simulink model "Adaptive_flux_observer_with_rotor_resistance_estimator"  (R2021a)
settings: Solver=FixedStepDiscrete  StartTime=0.0  StopTime=10.0  FixedStep=1e-5  RelTol=1e-3
undefined symbols (not defined in the file): DiscIntNeverNeededParam
settings Model: Creator=Mehra  LastModifiedBy=Mehra
settings SolverCC: ZeroCrossControl=DisableAll
settings DataIOCC: SaveOutput=off  SaveTime=off
settings GRTTargetCC: CombineOutputUpdateFcns=off  MatFileLogging=off

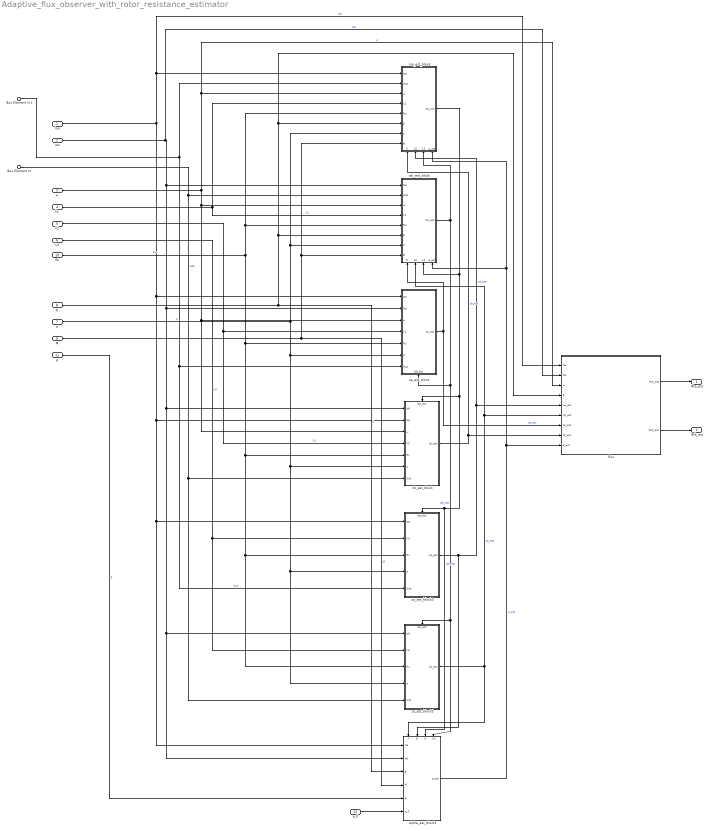
== system Adaptive_flux_observer_with_rotor_resistance_estimator ==
  Isa : Inport
  Isb : Inport  Port=2
  ω : Inport  Port=3
  k1 : Inport  Port=4
  k2 : Inport  Port=5
  k3 : Inport  Port=6
  σ : Inport  Port=7  OutDataTypeStr=double  PortDimensions=1
  β : Inport  Port=8  OutDataTypeStr=double  PortDimensions=1
  M : Inport  Port=9  OutDataTypeStr=double  PortDimensions=1
  Rs : Inport  Port=10
  g : Inport  Port=11
  α_0 : Inport  Port=12
  Bus Element In : Inport  Port=13  PortName=Uab  Element=Usb
  Bus Element In1 : Inport  Port=13  PortName=Uab  Element=Usa
  Isb_est_block : Subsystem
      settings: PortSchema="{\"entries\":[{\"content\":{\"sides\":[{\"content\":{\"connectorIds\":[\"In1\",\"In2\",\"In3\",\"In4\",\"In5\",\"In6\",\"In7\",\"In8\"]},\"type\":\"ConnectorPlacement.EquallySpacedRectSide\",\"uuid\":\"87550367-2c6c-480a-aae3-af00ec1c69b3\"},{\"content\":{\"connectorIds\":[\"Out1\"],\"side\":\"RIGHT\"},\"type\":\"ConnectorPlacement.EquallySpacedRectSide\",\"uuid\":\"4f526c6d-fa4b-4ae0-86ac-8e6f33c5fae1\"},{\"content\":{\"connectorIds\":[],\"side\":\"TOP\"},\"type\":\"ConnectorPlacement.EquallySpacedRectSide\",\"uuid\":\"2d7b9d3a-1034-4362-9035-011a628f41c9\"},{\"content\":{\"connectorIds\":[\"In9\",\"In10\",\"In11\",\"In12\"],\"side\":\"BOTTOM\"},\"type\":\"ConnectorPlacement.EquallySpacedRectSide\",\"uuid\":\"27bebb74-37d6-4f42-a6d1-29615f974c06\"}]},\"type\":\"ConnectorPlacement.EquallySpacedConnector\",\"uuid\":\"0c2c7644-fd75-4008-b344-0d549d52e423\"}],\"packageUris\":[\"http://schema.mathworks.com/mf0/Connector/R2020b\"],\"version\":\"1.0\"}"
  alpha_est_block1 : Subsystem
      settings: PortSchema="{\"entries\":[{\"content\":{\"sides\":[{\"content\":{\"connectorIds\":[\"In1\",\"In2\",\"In3\",\"In4\",\"In5\",\"In6\"]},\"type\":\"ConnectorPlacement.EquallySpacedRectSide\",\"uuid\":\"13ad627c-6f07-4cec-b595-5beaa6b2cc7c\"},{\"content\":{\"connectorIds\":[\"Out1\"],\"side\":\"RIGHT\"},\"type\":\"ConnectorPlacement.EquallySpacedRectSide\",\"uuid\":\"277076a7-856b-4e3b-b26b-d287057d48dc\"},{\"content\":{\"connectorIds\":[\"In7\",\"In8\",\"In9\",\"In10\"],\"side\":\"TOP\"},\"type\":\"ConnectorPlacement.EquallySpacedRectSide\",\"uuid\":\"ff90b138-b04e-44ba-87a2-7f09928b1812\"},{\"content\":{\"connectorIds\":[],\"side\":\"BOTTOM\"},\"type\":\"ConnectorPlacement.EquallySpacedRectSide\",\"uuid\":\"47c98a3f-b8ed-4eae-8b18-f11cd62e73ac\"}]},\"type\":\"ConnectorPlacement.EquallySpacedConnector\",\"uuid\":\"bcf44069-4ce9-4b3f-954c-53de8c0b8283\"}],\"packageUris\":[\"http://schema.mathworks.com/mf0/Connector/R2020b\"],\"version\":\"1.0\"}"
  flux : Subsystem
  isa_est_block : Subsystem
      settings: PortSchema="{\"entries\":[{\"content\":{\"sides\":[{\"content\":{\"connectorIds\":[\"In1\",\"In2\",\"In3\",\"In4\",\"In5\",\"In6\",\"In7\",\"In8\"]},\"type\":\"ConnectorPlacement.EquallySpacedRectSide\",\"uuid\":\"87550367-2c6c-480a-aae3-af00ec1c69b3\"},{\"content\":{\"connectorIds\":[\"Out1\"],\"side\":\"RIGHT\"},\"type\":\"ConnectorPlacement.EquallySpacedRectSide\",\"uuid\":\"4f526c6d-fa4b-4ae0-86ac-8e6f33c5fae1\"},{\"content\":{\"connectorIds\":[],\"side\":\"TOP\"},\"type\":\"ConnectorPlacement.EquallySpacedRectSide\",\"uuid\":\"2d7b9d3a-1034-4362-9035-011a628f41c9\"},{\"content\":{\"connectorIds\":[\"In9\",\"In10\",\"In11\",\"In12\"],\"side\":\"BOTTOM\"},\"type\":\"ConnectorPlacement.EquallySpacedRectSide\",\"uuid\":\"27bebb74-37d6-4f42-a6d1-29615f974c06\"}]},\"type\":\"ConnectorPlacement.EquallySpacedConnector\",\"uuid\":\"0c2c7644-fd75-4008-b344-0d549d52e423\"}],\"packageUris\":[\"http://schema.mathworks.com/mf0/Connector/R2020b\"],\"version\":\"1.0\"}"
  za_est_block : Subsystem
      settings: PortSchema="{\"entries\":[{\"content\":{\"sides\":[{\"content\":{\"connectorIds\":[\"In1\",\"In2\",\"In3\",\"In4\",\"In5\",\"In6\",\"In7\"]},\"type\":\"ConnectorPlacement.EquallySpacedRectSide\",\"uuid\":\"13ad627c-6f07-4cec-b595-5beaa6b2cc7c\"},{\"content\":{\"connectorIds\":[\"Out1\"],\"side\":\"RIGHT\"},\"type\":\"ConnectorPlacement.EquallySpacedRectSide\",\"uuid\":\"277076a7-856b-4e3b-b26b-d287057d48dc\"},{\"content\":{\"connectorIds\":[],\"side\":\"TOP\"},\"type\":\"ConnectorPlacement.EquallySpacedRectSide\",\"uuid\":\"ff90b138-b04e-44ba-87a2-7f09928b1812\"},{\"content\":{\"connectorIds\":[\"In8\"],\"side\":\"BOTTOM\"},\"type\":\"ConnectorPlacement.EquallySpacedRectSide\",\"uuid\":\"47c98a3f-b8ed-4eae-8b18-f11cd62e73ac\"}]},\"type\":\"ConnectorPlacement.EquallySpacedConnector\",\"uuid\":\"bcf44069-4ce9-4b3f-954c-53de8c0b8283\"}],\"packageUris\":[\"http://schema.mathworks.com/mf0/Connector/R2020b\"],\"version\":\"1.0\"}"
  za_est_block2 : Subsystem
      settings: PortSchema="{\"entries\":[{\"content\":{\"sides\":[{\"content\":{\"connectorIds\":[\"In1\",\"In2\",\"In3\",\"In4\",\"In5\"]},\"type\":\"ConnectorPlacement.EquallySpacedRectSide\",\"uuid\":\"13ad627c-6f07-4cec-b595-5beaa6b2cc7c\"},{\"content\":{\"connectorIds\":[\"Out1\"],\"side\":\"RIGHT\"},\"type\":\"ConnectorPlacement.EquallySpacedRectSide\",\"uuid\":\"277076a7-856b-4e3b-b26b-d287057d48dc\"},{\"content\":{\"connectorIds\":[\"In6\"],\"side\":\"TOP\"},\"type\":\"ConnectorPlacement.EquallySpacedRectSide\",\"uuid\":\"ff90b138-b04e-44ba-87a2-7f09928b1812\"},{\"content\":{\"connectorIds\":[],\"side\":\"BOTTOM\"},\"type\":\"ConnectorPlacement.EquallySpacedRectSide\",\"uuid\":\"47c98a3f-b8ed-4eae-8b18-f11cd62e73ac\"}]},\"type\":\"ConnectorPlacement.EquallySpacedConnector\",\"uuid\":\"bcf44069-4ce9-4b3f-954c-53de8c0b8283\"}],\"packageUris\":[\"http://schema.mathworks.com/mf0/Connector/R2020b\"],\"version\":\"1.0\"}"
  za_est_block3 : Subsystem
      settings: PortSchema="{\"entries\":[{\"content\":{\"sides\":[{\"content\":{\"connectorIds\":[\"In1\",\"In2\",\"In3\",\"In4\",\"In5\"]},\"type\":\"ConnectorPlacement.EquallySpacedRectSide\",\"uuid\":\"13ad627c-6f07-4cec-b595-5beaa6b2cc7c\"},{\"content\":{\"connectorIds\":[\"Out1\"],\"side\":\"RIGHT\"},\"type\":\"ConnectorPlacement.EquallySpacedRectSide\",\"uuid\":\"277076a7-856b-4e3b-b26b-d287057d48dc\"},{\"content\":{\"connectorIds\":[\"In6\"],\"side\":\"TOP\"},\"type\":\"ConnectorPlacement.EquallySpacedRectSide\",\"uuid\":\"ff90b138-b04e-44ba-87a2-7f09928b1812\"},{\"content\":{\"connectorIds\":[],\"side\":\"BOTTOM\"},\"type\":\"ConnectorPlacement.EquallySpacedRectSide\",\"uuid\":\"47c98a3f-b8ed-4eae-8b18-f11cd62e73ac\"}]},\"type\":\"ConnectorPlacement.EquallySpacedConnector\",\"uuid\":\"bcf44069-4ce9-4b3f-954c-53de8c0b8283\"}],\"packageUris\":[\"http://schema.mathworks.com/mf0/Connector/R2020b\"],\"version\":\"1.0\"}"
  zb_est_block : Subsystem
      settings: PortSchema="{\"entries\":[{\"content\":{\"sides\":[{\"content\":{\"connectorIds\":[\"In1\",\"In2\",\"In3\",\"In4\",\"In5\",\"In6\",\"In7\"]},\"type\":\"ConnectorPlacement.EquallySpacedRectSide\",\"uuid\":\"13ad627c-6f07-4cec-b595-5beaa6b2cc7c\"},{\"content\":{\"connectorIds\":[\"Out1\"],\"side\":\"RIGHT\"},\"type\":\"ConnectorPlacement.EquallySpacedRectSide\",\"uuid\":\"277076a7-856b-4e3b-b26b-d287057d48dc\"},{\"content\":{\"connectorIds\":[\"In8\"],\"side\":\"TOP\"},\"type\":\"ConnectorPlacement.EquallySpacedRectSide\",\"uuid\":\"ff90b138-b04e-44ba-87a2-7f09928b1812\"},{\"content\":{\"connectorIds\":[],\"side\":\"BOTTOM\"},\"type\":\"ConnectorPlacement.EquallySpacedRectSide\",\"uuid\":\"47c98a3f-b8ed-4eae-8b18-f11cd62e73ac\"}]},\"type\":\"ConnectorPlacement.EquallySpacedConnector\",\"uuid\":\"bcf44069-4ce9-4b3f-954c-53de8c0b8283\"}],\"packageUris\":[\"http://schema.mathworks.com/mf0/Connector/R2020b\"],\"version\":\"1.0\"}"
  Ψra_est : Outport
  Ψrb_est : Outport  Port=2
  wires:
  Isa/1 -> flux/1(Isa), isa_est_block/1(Isa), alpha_est_block1/1(Isa), za_est_block3/1(Isa), zb_est_block/2(Isa), za_est_block/1(Isa)  "Isa"
  Bus Element In1/1 -> za_est_block3/5(Usa), za_est_block/7(Usa), isa_est_block/2(Usa)  "Usa"
  ω/1 -> zb_est_block/3(ω), za_est_block/3(ω), Isb_est_block/3(ω), isa_est_block/3(ω), flux/3(ω)  "ω"
  k1/1 -> Isb_est_block/4(k1), isa_est_block/4(k1)  "k1"
  Rs/1 -> za_est_block2/3(Rs), za_est_block3/3(Rs), zb_est_block/5(Rs), za_est_block/5(Rs), Isb_est_block/5(Rs), isa_est_block/5(Rs)  "Rs"
  β/1 -> flux/4(β), isa_est_block/6(β), Isb_est_block/6(β), alpha_est_block1/3(β)  "β"
  σ/1 -> za_est_block2/4(σ), za_est_block3/4(σ), zb_est_block/6(σ), za_est_block/6(σ), Isb_est_block/7(σ), isa_est_block/7(σ)  "σ"
  M/1 -> alpha_est_block1/4(M), isa_est_block/8(M), Isb_est_block/8(M)  "M"
  isa_est_block/1(Isa_est) -> Isb_est_block/11(Isa_est), zb_est_block/8(Isa_est), alpha_est_block1/9(Isa_est), za_est_block3/6(Isa_est)  "Isa_est"
  Isb/1 -> flux/2(Isb), alpha_est_block1/2(Isb), za_est_block2/1(Isb), zb_est_block/1(Isb), za_est_block/2(Isb), Isb_est_block/1(Isb)  "Isb"
  Bus Element In/1 -> za_est_block2/5(Usb), zb_est_block/7(Usb), Isb_est_block/2(Usb)  "Usb"
  Isb_est_block/1(Isb_est) -> za_est_block/8(Isb_est), alpha_est_block1/10(Isb_est), za_est_block2/6(Isb_est), isa_est_block/11(Isb_est)  "Isb_est"
  za_est_block/1(za_est) -> flux/7(za_est), Isb_est_block/9(za_est)  "za_est"
  k2/1 -> zb_est_block/4(k2), za_est_block/4(k2)  "k2"
  zb_est_block/1(zb_est) -> isa_est_block/9(zb_est), flux/8(zb_est)  "zb_est"
  k3/1 -> za_est_block2/2(k3), za_est_block3/2(k3)  "k3"
  za_est_block3/1(ηa_est) -> flux/5(ηa_est), isa_est_block/10(ηa_est), alpha_est_block1/8(ηa_est)  "ηa_est"
  za_est_block2/1(ηb_est) -> flux/6(ηb_est), Isb_est_block/10(ηb_est), alpha_est_block1/7(ηb_est)  "ηb_est"
  g/1 -> alpha_est_block1/5(g)  "g"
  alpha_est_block1/1(α_est) -> flux/9(α_est), isa_est_block/12(α_est), Isb_est_block/12(α_est)  "α_est"
  flux/1(Ψra_est) -> Ψra_est/1
  flux/2(Ψrb_est) -> Ψrb_est/1
  α_0/1 -> alpha_est_block1/6(α_0)

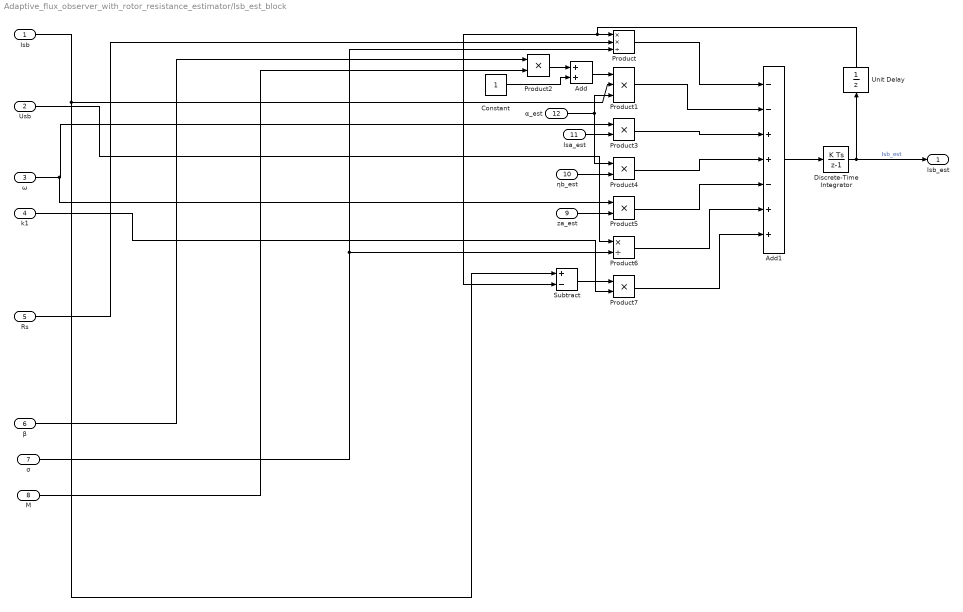
== system Adaptive_flux_observer_with_rotor_resistance_estimator/Isb_est_block ==
  Isb : Inport
  Usb : Inport  Port=2
  ω : Inport  Port=3
  k1 : Inport  Port=4
  Rs : Inport  Port=5
  β : Inport  Port=6
  σ : Inport  Port=7
  M : Inport  Port=8
  za_est : Inport  Port=9
  ηb_est : Inport  Port=10
  Isa_est : Inport  Port=11
  α_est : Inport  Port=12
  Add : Sum
  Add1 : Sum  Inputs=--++-++
  Constant : Constant
  Discrete-Time Integrator : DiscreteIntegrator  SampleTime=-1  ICPrevOutput=DiscIntNeverNeededParam  ICPrevScaledInput=DiscIntNeverNeededParam
  Product : Product  Inputs=**/
  Product1 : Product  Inputs=3
  Product{2..5,7} (5 alike) : Product
  Product6 : Product  Inputs=*/
  Subtract : Sum  Inputs=+-
  Unit Delay : UnitDelay  SampleTime=-1  HasFrameUpgradeWarning=on
  Isb_est : Outport
  wires:
  Product7/1 -> Add1/7
  β/1 -> Product2/1
  Product1/1 -> Add1/2
  Constant/1 -> Add/2
  Product2/1 -> Add/1
  Discrete-Time Integrator/1 -> Isb_est/1, Unit Delay/1  "Isb_est"
  Product6/1 -> Add1/6
  Add/1 -> Product1/1
  Subtract/1 -> Product7/1
  Product3/1 -> Add1/3
  Product5/1 -> Add1/5
  ηb_est/1 -> Product4/2
  σ/1 -> Product/3, Product6/2
  ω/1 -> Product5/1, Product3/1
  Isb/1 -> Subtract/1, Product1/2
  Product4/1 -> Add1/4
  Add1/1 -> Discrete-Time Integrator/1
  Product/1 -> Add1/1
  Rs/1 -> Product/2
  M/1 -> Product2/2
  α_est/1 -> Product1/3, Product4/1
  Isa_est/1 -> Product3/2
  Usb/1 -> Product6/1
  za_est/1 -> Product5/2
  k1/1 -> Product7/2
  Unit Delay/1 -> Subtract/2, Product/1

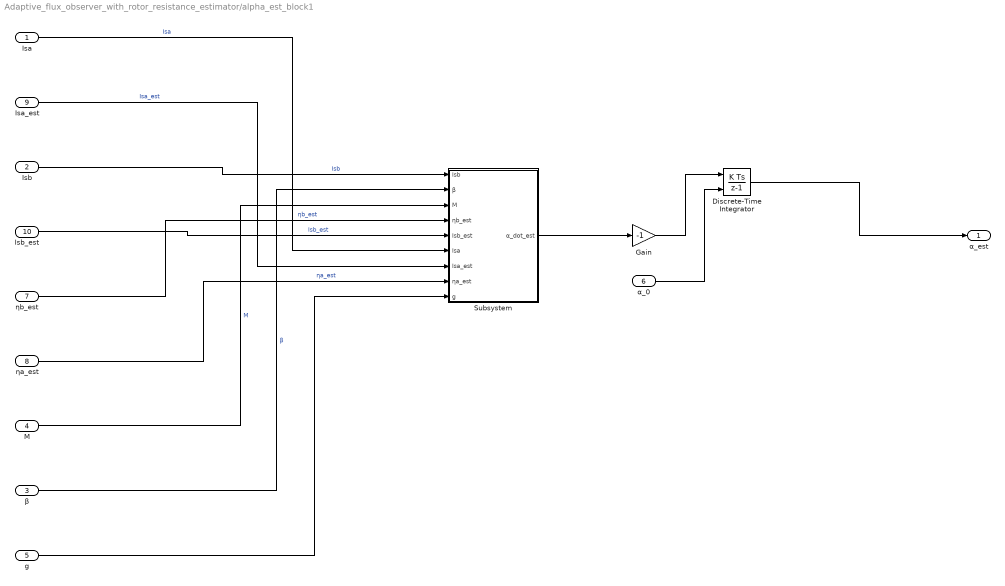
== system Adaptive_flux_observer_with_rotor_resistance_estimator/alpha_est_block1 ==
  Isa : Inport
  Isb : Inport  Port=2
  β : Inport  Port=3
  M : Inport  Port=4
  g : Inport  Port=5
  α_0 : Inport  Port=6
  ηb_est : Inport  Port=7
  ηa_est : Inport  Port=8
  Isa_est : Inport  Port=9
  Isb_est : Inport  Port=10
  Discrete-Time Integrator : DiscreteIntegrator  InitialConditionSource=external  SampleTime=-1  ICPrevOutput=DiscIntNeverNeededParam  ICPrevScaledInput=DiscIntNeverNeededParam
  Gain : Gain  Gain=-1
  Subsystem : Subsystem
  α_est : Outport
  wires:
  Isb/1 -> Subsystem/1(Isb)  "Isb"
  β/1 -> Subsystem/2(β)  "β"
  M/1 -> Subsystem/3(M)  "M"
  ηb_est/1 -> Subsystem/4(ηb_est)  "ηb_est"
  Isb_est/1 -> Subsystem/5(Isb_est)  "Isb_est"
  Isa/1 -> Subsystem/6(Isa)  "Isa"
  Isa_est/1 -> Subsystem/7(Isa_est)  "Isa_est"
  ηa_est/1 -> Subsystem/8(ηa_est)  "ηa_est"
  g/1 -> Subsystem/9(g)
  Discrete-Time Integrator/1 -> α_est/1
  Subsystem/1(α_dot_est) -> Gain/1
  Gain/1 -> Discrete-Time Integrator/1
  α_0/1 -> Discrete-Time Integrator/2

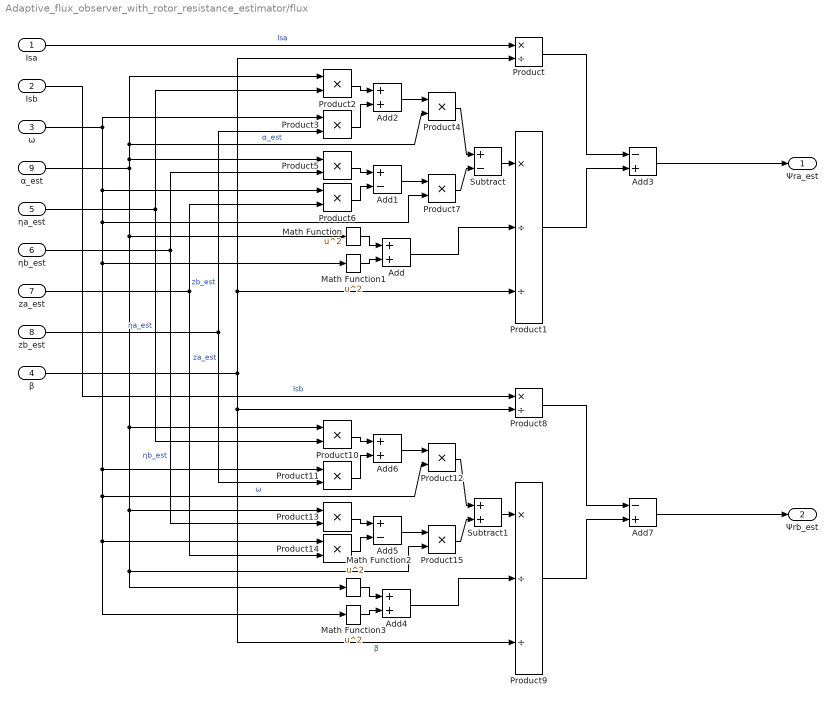
== system Adaptive_flux_observer_with_rotor_resistance_estimator/flux ==
  Isa : Inport
  Isb : Inport  Port=2
  ω : Inport  Port=3
  β : Inport  Port=4
  ηa_est : Inport  Port=5
  ηb_est : Inport  Port=6
  za_est : Inport  Port=7
  zb_est : Inport  Port=8
  α_est : Inport  Port=9
  Add{,2,4,6} (4 alike) : Sum
  Add1 : Sum  Inputs=+-
  Add3 : Sum  Inputs=-+
  Add5 : Sum  Inputs=+-
  Add7 : Sum  Inputs=-+
  Math Function{,1..3} (4 alike) : Math  Operator=square  SaturateOnIntegerOverflow=on
  Product : Product  Inputs=*/
  Product1 : Product  Inputs=*//
  Product{2..7,10..15} (12 alike) : Product
  Product8 : Product  Inputs=*/
  Product9 : Product  Inputs=*//
  Subtract : Sum  Inputs=+-
  Subtract1 : Sum
  Ψra_est : Outport
  Ψrb_est : Outport  Port=2
  wires:
  Isa/1 -> Product/1  "Isa"
  β/1 -> Product9/3, Product8/2, Product/2, Product1/3  "β"
  α_est/1 -> Product5/1, Product4/2, Product2/1, Product10/1, Product15/2, Math Function2/1, Product13/1, Math Function/1  "α_est"
  Math Function/1 -> Add/1
  Math Function1/1 -> Add/2
  Add/1 -> Product1/2
  ω/1 -> Product6/1, Product7/2, Product12/2, Math Function3/1, Product14/1, Product11/1, Math Function1/1, Product3/1  "ω"
  ηa_est/1 -> Product10/2, Product2/2  "ηa_est"
  zb_est/1 -> Product11/2, Product3/2  "zb_est"
  Product2/1 -> Add2/1
  Product3/1 -> Add2/2
  Add2/1 -> Product4/1
  Subtract/1 -> Product1/1
  Product4/1 -> Subtract/1
  Add1/1 -> Product7/1
  Product6/1 -> Add1/2
  Product5/1 -> Add1/1
  Product7/1 -> Subtract/2
  ηb_est/1 -> Product13/2, Product5/2  "ηb_est"
  za_est/1 -> Product14/2, Product6/2  "za_est"
  Product/1 -> Add3/1
  Product1/1 -> Add3/2
  Add3/1 -> Ψra_est/1
  Product9/1 -> Add7/2
  Add4/1 -> Product9/2
  Math Function2/1 -> Add4/1
  Add6/1 -> Product12/1
  Product12/1 -> Subtract1/1
  Product15/1 -> Subtract1/2
  Product8/1 -> Add7/1
  Product14/1 -> Add5/2
  Product13/1 -> Add5/1
  Add5/1 -> Product15/1
  Subtract1/1 -> Product9/1
  Product11/1 -> Add6/2
  Math Function3/1 -> Add4/2
  Product10/1 -> Add6/1
  Isb/1 -> Product8/1  "Isb"
  Add7/1 -> Ψrb_est/1

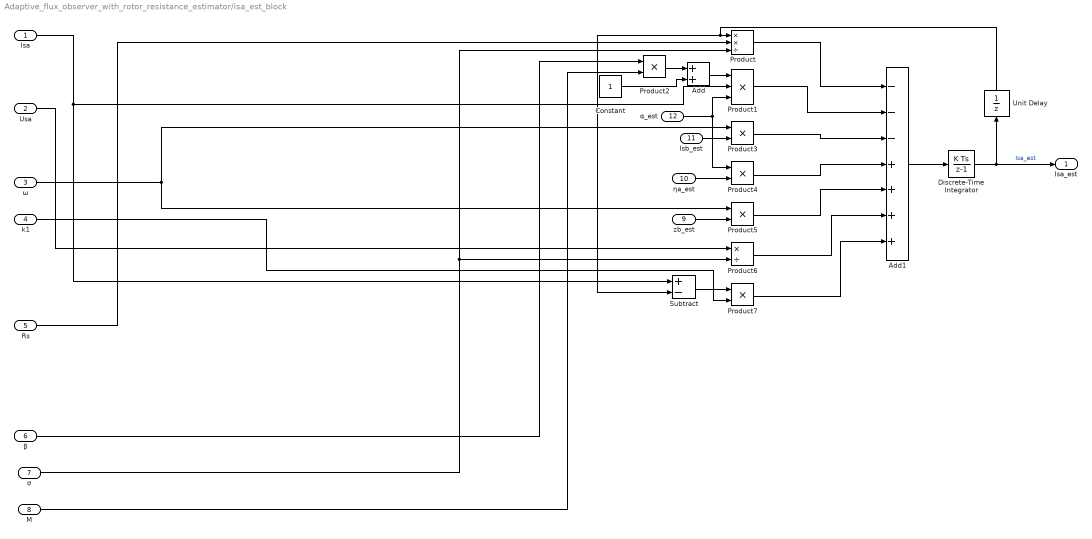
== system Adaptive_flux_observer_with_rotor_resistance_estimator/isa_est_block ==
  Isa : Inport
  Usa : Inport  Port=2
  ω : Inport  Port=3
  k1 : Inport  Port=4
  Rs : Inport  Port=5
  β : Inport  Port=6
  σ : Inport  Port=7
  M : Inport  Port=8
  zb_est : Inport  Port=9
  ηa_est : Inport  Port=10
  Isb_est : Inport  Port=11
  α_est : Inport  Port=12
  Add : Sum
  Add1 : Sum  Inputs=---++++
  Constant : Constant
  Discrete-Time Integrator : DiscreteIntegrator  SampleTime=-1  ICPrevOutput=DiscIntNeverNeededParam  ICPrevScaledInput=DiscIntNeverNeededParam
  Product : Product  Inputs=**/
  Product1 : Product  Inputs=3
  Product{2..5,7} (5 alike) : Product
  Product6 : Product  Inputs=*/
  Subtract : Sum  Inputs=+-
  Unit Delay : UnitDelay  SampleTime=-1  HasFrameUpgradeWarning=on
  Isa_est : Outport
  wires:
  Product7/1 -> Add1/7
  β/1 -> Product2/1
  Product1/1 -> Add1/2
  Constant/1 -> Add/2
  Product2/1 -> Add/1
  Discrete-Time Integrator/1 -> Unit Delay/1, Isa_est/1  "Isa_est"
  Product6/1 -> Add1/6
  Add/1 -> Product1/1
  Subtract/1 -> Product7/1
  Product3/1 -> Add1/3
  Product5/1 -> Add1/5
  ηa_est/1 -> Product4/2
  σ/1 -> Product/3, Product6/2
  ω/1 -> Product5/1, Product3/1
  Isa/1 -> Subtract/1, Product1/2
  Product4/1 -> Add1/4
  Add1/1 -> Discrete-Time Integrator/1
  Product/1 -> Add1/1
  Rs/1 -> Product/2
  M/1 -> Product2/2
  α_est/1 -> Product1/3, Product4/1
  Isb_est/1 -> Product3/2
  Usa/1 -> Product6/1
  zb_est/1 -> Product5/2
  k1/1 -> Product7/2
  Unit Delay/1 -> Subtract/2, Product/1

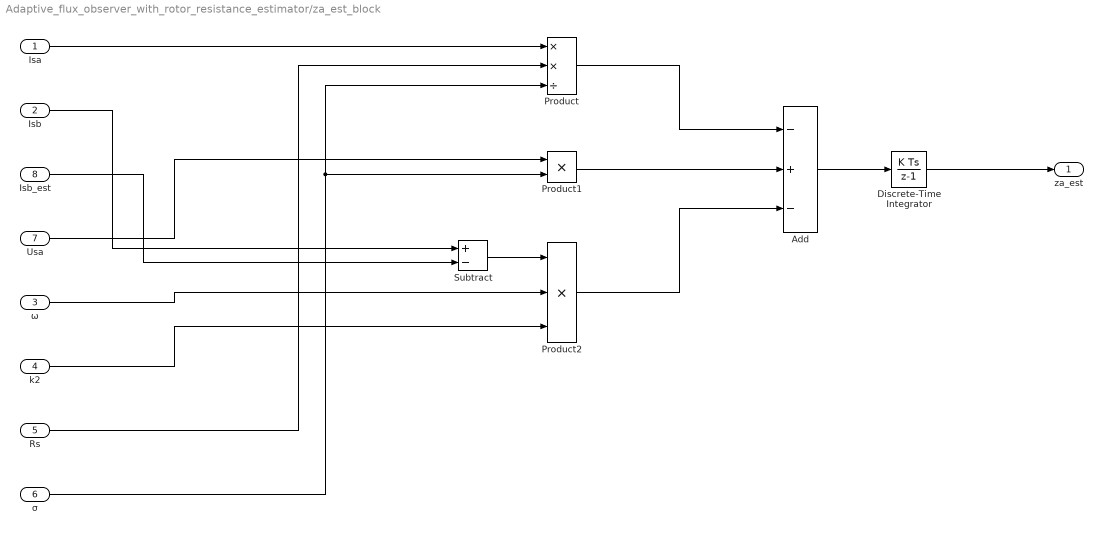
== system Adaptive_flux_observer_with_rotor_resistance_estimator/za_est_block ==
  Isa : Inport
  Isb : Inport  Port=2
  ω : Inport  Port=3
  k2 : Inport  Port=4
  Rs : Inport  Port=5
  σ : Inport  Port=6
  Usa : Inport  Port=7
  Isb_est : Inport  Port=8
  Add : Sum  Inputs=-+-
  Discrete-Time Integrator : DiscreteIntegrator  SampleTime=-1  ICPrevOutput=DiscIntNeverNeededParam  ICPrevScaledInput=DiscIntNeverNeededParam
  Product : Product  Inputs=**/
  Product1 : Product
  Product2 : Product  Inputs=***
  Subtract : Sum  Inputs=+-
  za_est : Outport
  wires:
  Isa/1 -> Product/1
  Rs/1 -> Product/2
  σ/1 -> Product1/2, Product/3
  Usa/1 -> Product1/1
  Subtract/1 -> Product2/1
  Isb/1 -> Subtract/1
  Isb_est/1 -> Subtract/2
  ω/1 -> Product2/2
  k2/1 -> Product2/3
  Product/1 -> Add/1
  Product1/1 -> Add/2
  Product2/1 -> Add/3
  Add/1 -> Discrete-Time Integrator/1
  Discrete-Time Integrator/1 -> za_est/1

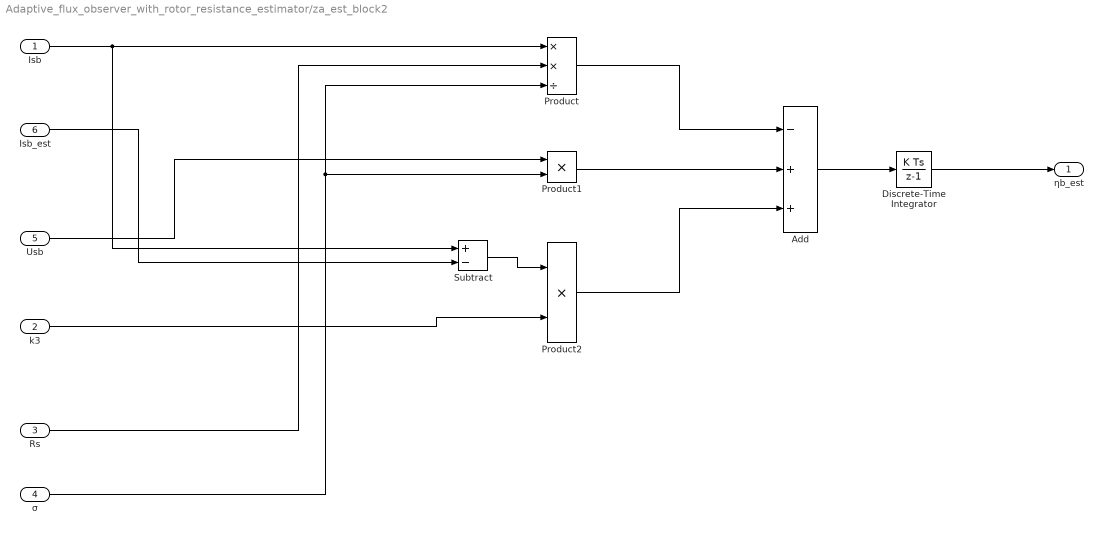
== system Adaptive_flux_observer_with_rotor_resistance_estimator/za_est_block2 ==
  Isb : Inport
  k3 : Inport  Port=2
  Rs : Inport  Port=3
  σ : Inport  Port=4
  Usb : Inport  Port=5
  Isb_est : Inport  Port=6
  Add : Sum  Inputs=-++
  Discrete-Time Integrator : DiscreteIntegrator  SampleTime=-1  ICPrevOutput=DiscIntNeverNeededParam  ICPrevScaledInput=DiscIntNeverNeededParam
  Product : Product  Inputs=**/
  Product1 : Product
  Product2 : Product
  Subtract : Sum  Inputs=+-
  ηb_est : Outport
  wires:
  Rs/1 -> Product/2
  σ/1 -> Product1/2, Product/3
  Usb/1 -> Product1/1
  Subtract/1 -> Product2/1
  Isb/1 -> Subtract/1, Product/1
  Isb_est/1 -> Subtract/2
  Product/1 -> Add/1
  Product1/1 -> Add/2
  Product2/1 -> Add/3
  Add/1 -> Discrete-Time Integrator/1
  Discrete-Time Integrator/1 -> ηb_est/1
  k3/1 -> Product2/2

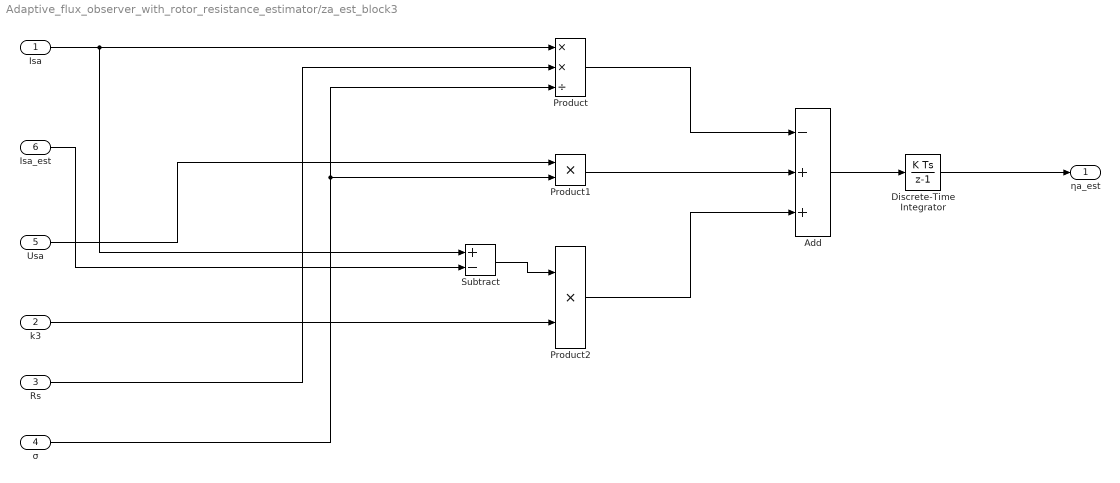
== system Adaptive_flux_observer_with_rotor_resistance_estimator/za_est_block3 ==
  Isa : Inport
  k3 : Inport  Port=2
  Rs : Inport  Port=3
  σ : Inport  Port=4
  Usa : Inport  Port=5
  Isa_est : Inport  Port=6
  Add : Sum  Inputs=-++
  Discrete-Time Integrator : DiscreteIntegrator  SampleTime=-1  ICPrevOutput=DiscIntNeverNeededParam  ICPrevScaledInput=DiscIntNeverNeededParam
  Product : Product  Inputs=**/
  Product1 : Product
  Product2 : Product
  Subtract : Sum  Inputs=+-
  ηa_est : Outport
  wires:
  Isa/1 -> Subtract/1, Product/1
  Rs/1 -> Product/2
  σ/1 -> Product1/2, Product/3
  Usa/1 -> Product1/1
  Subtract/1 -> Product2/1
  Isa_est/1 -> Subtract/2
  Product/1 -> Add/1
  Product1/1 -> Add/2
  Product2/1 -> Add/3
  Add/1 -> Discrete-Time Integrator/1
  Discrete-Time Integrator/1 -> ηa_est/1
  k3/1 -> Product2/2

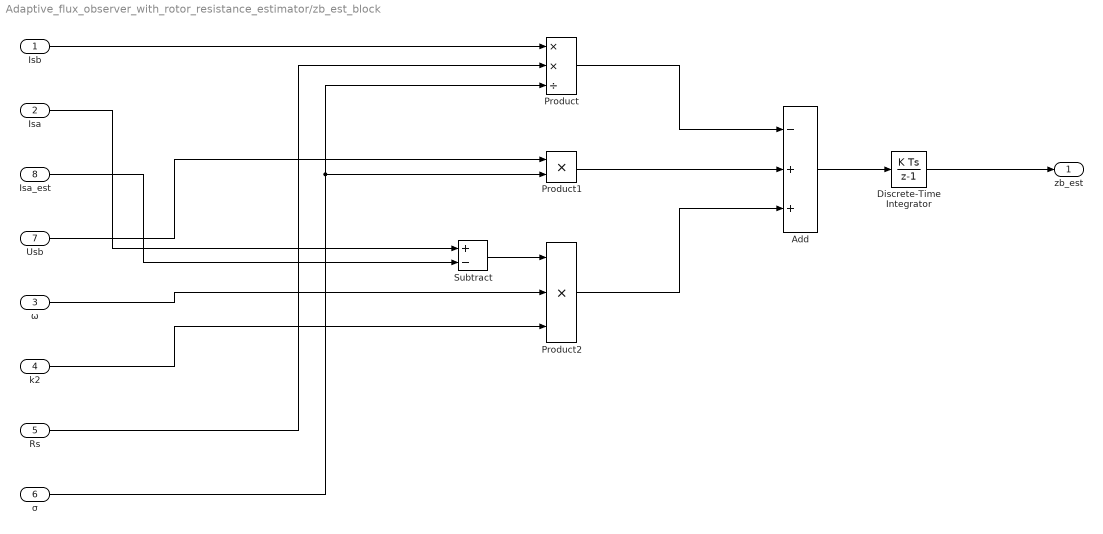
== system Adaptive_flux_observer_with_rotor_resistance_estimator/zb_est_block ==
  Isb : Inport
  Isa : Inport  Port=2
  ω : Inport  Port=3
  k2 : Inport  Port=4
  Rs : Inport  Port=5
  σ : Inport  Port=6
  Usb : Inport  Port=7
  Isa_est : Inport  Port=8
  Add : Sum  Inputs=-++
  Discrete-Time Integrator : DiscreteIntegrator  SampleTime=-1  ICPrevOutput=DiscIntNeverNeededParam  ICPrevScaledInput=DiscIntNeverNeededParam
  Product : Product  Inputs=**/
  Product1 : Product
  Product2 : Product  Inputs=***
  Subtract : Sum  Inputs=+-
  zb_est : Outport
  wires:
  Isb/1 -> Product/1
  Rs/1 -> Product/2
  σ/1 -> Product1/2, Product/3
  Usb/1 -> Product1/1
  Subtract/1 -> Product2/1
  Isa/1 -> Subtract/1
  Isa_est/1 -> Subtract/2
  ω/1 -> Product2/2
  k2/1 -> Product2/3
  Product/1 -> Add/1
  Product1/1 -> Add/2
  Product2/1 -> Add/3
  Add/1 -> Discrete-Time Integrator/1
  Discrete-Time Integrator/1 -> zb_est/1

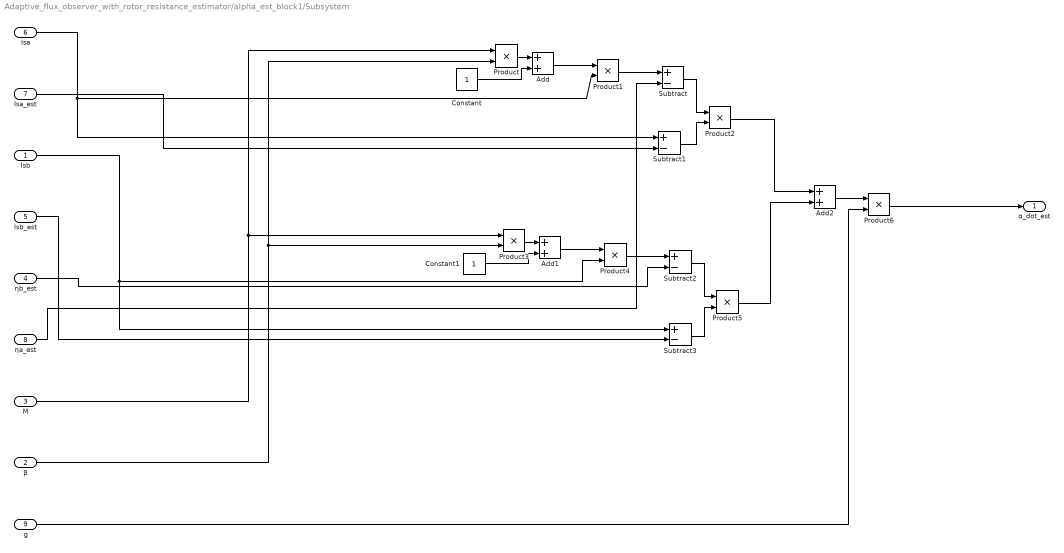
== system Adaptive_flux_observer_with_rotor_resistance_estimator/alpha_est_block1/Subsystem ==
  Isb : Inport
  β : Inport  Port=2
  M : Inport  Port=3
  ηb_est : Inport  Port=4
  Isb_est : Inport  Port=5
  Isa : Inport  Port=6
  Isa_est : Inport  Port=7
  ηa_est : Inport  Port=8
  g : Inport  Port=9
  Add : Sum
  Add1 : Sum
  Add2 : Sum
  Constant : Constant
  Constant1 : Constant
  Product{,1..6} (7 alike) : Product
  Subtract{,1..3} (4 alike) : Sum  Inputs=+-
  α_dot_est : Outport
  wires:
  Product5/1 -> Add2/2
  Isa/1 -> Subtract1/1, Product1/2
  Product2/1 -> Add2/1
  Subtract/1 -> Product2/1
  Isa_est/1 -> Subtract1/2
  ηb_est/1 -> Subtract2/2
  Product4/1 -> Subtract2/1
  M/1 -> Product3/1, Product/1
  Product/1 -> Add/1
  Subtract3/1 -> Product5/2
  β/1 -> Product/2, Product3/2
  ηa_est/1 -> Subtract/2
  Constant1/1 -> Add1/2
  Subtract1/1 -> Product2/2
  Product3/1 -> Add1/1
  Add1/1 -> Product4/1
  Isb/1 -> Product4/2, Subtract3/1
  Subtract2/1 -> Product5/1
  Add/1 -> Product1/1
  Isb_est/1 -> Subtract3/2
  Constant/1 -> Add/2
  Product1/1 -> Subtract/1
  Add2/1 -> Product6/1
  g/1 -> Product6/2
  Product6/1 -> α_dot_est/1
